simulink model "VbyFSpeedControl"  (R2017b)
settings: Solver=VariableStepAuto  StartTime=0.0  StopTime=10  MaxStep=1e-4  RelTol=1e-3
undefined symbols (not defined in the file): sigbuilder_block
libraries: powerlib x7, powerlib_meascontrol x1
settings Model: Creator=u4eee15106  LastModifiedBy=india
settings OptimizationCC: LifeSpan=inf
settings DebuggingCC: SFExecutionAtInitializationDiag=none
settings CodeAppCC: StateflowObjectComments=on

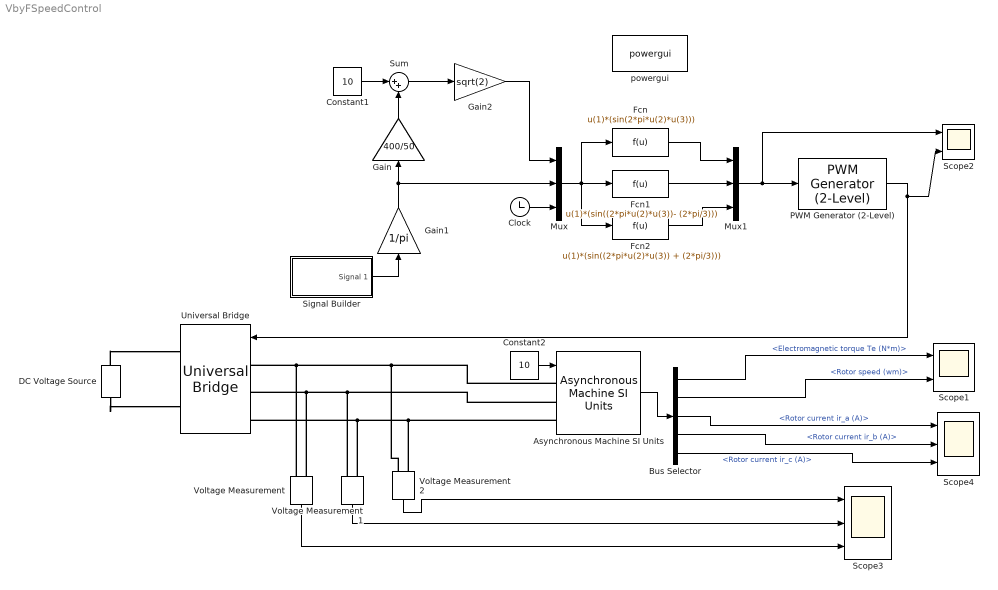
== system VbyFSpeedControl ==
  Asynchronous Machine SI Units : powerlib/Machines/Asynchronous Machine SI Units  RotorType=Squirrel-cage  PresetModel="15:  5.4 HP (4KW)   400 V  50Hz 1430 RPM"  MechanicalLoad=Torque Tm  ShowDetailedParameters=on  ReferenceFrame=Rotor  Units=SI  MeasurementBus=off  NominalParameters=[4000 400 50]  Stator=[1.405 0.005839]  Rotor=[1.395 0.005839]  Cage1=[0.4155 0.002066]  Cage2=[0.4168 0.0003495]  Lm=0.1722  Mechanical=[0.0131 0.002985 2]  PolePairs=2  InitialConditions=[0 0 0 0 0 0 0 0]  SimulateSaturation=off  Saturation=[14.03593122, 27.81365428, 53.79336849, 72.68890987, 97.98006896, 148.6815601, 215.7428561, 302.9841135, 428.7778367 ; 230, 322, 414, 460, 506, 552, 598, 644, 690]  LoadFlowParameters=1492000  TsPowergui=0  TsBlock=-1  IterativeModel=Trapezoidal non iterative  IterativeDiscreteModel=Trapezoidal non iterative  Pmec=1.492e+006
  Bus Selector : BusSelector  OutputSignals=Mechanical.Electromagnetic torque Te (N*m),Mechanical.Rotor speed (wm),Rotor measurements.Rotor current ir_a (A),Rotor measurements.Rotor current ir_b (A),Rotor measurements.Rotor current ir_c (A)
  Clock : Clock
  Constant1 : Constant  Value=10
  Constant2 : Constant  Value=10
  DC Voltage Source : powerlib/Electrical Sources/DC Voltage Source  Amplitude=415  Measurements=None
  Fcn : Fcn  Expr=u(1)*(sin(2*pi*u(2)*u(3)))
  Fcn1 : Fcn  Expr=u(1)*(sin((2*pi*u(2)*u(3))- (2*pi/3)))
  Fcn2 : Fcn  Expr=u(1)*(sin((2*pi*u(2)*u(3)) + (2*pi/3)))
  Gain : Gain  Gain=400/50
  Gain1 : Gain  Gain=1/pi
  Gain2 : Gain  Gain=sqrt(2)
  Mux : Mux  Inputs=3
  Mux1 : Mux  Inputs=3
  PWM Generator (2-Level) : powerlib_meascontrol/Pulse & Signal Generators/PWM Generator (2-Level)  ModulatorType=Three-phase bridge (6 pulses)  ModulatorMode=Unsynchronized  Fc=27*50  Pc=90  nF=27  MinMax="[ -1  1 ]"  SamplingTechnique=Natural  ModulatingSignals=off  m=0.8  Freq=60  Phase=0  Ts=0  ShowCarrierOutport=off
      settings: SourceProductName=Simscape Power Systems
  Scope1 : Scope  NumInputPorts=2
  Scope2 : Scope  NumInputPorts=2
  Scope3 : Scope  NumInputPorts=3
  Scope4 : Scope  NumInputPorts=3
  Signal Builder : Subsystem  Tag=STV Subsys  LoadFcn=sigbuilder_block('load');  StartFcn=sigbuilder_block('start');  StopFcn=sigbuilder_block('stop');  ClipboardFcn=sigbuilder_block('clipboard');  mask(Sigbuilder block){tuvar=[0:10]}
      mask help: Simulink:masks:SigbuilderBlock_MD
      mask init:
      | if ~strcmp(get_param(bdroot(gcbh),'SimulationStatus'),'stopped') tuvar = sigbuilder_block('maskInit'); end
      settings: CopyFcn=sigbuilder_block('copy');  DeleteFcn=sigbuilder_block('delete');  ModelCloseFcn=sigbuilder_block('modelClose');  PreSaveFcn=sigbuilder_block('preSave');  PauseFcn=sigbuilder_block('pause');  ContinueFcn=sigbuilder_block('continue');  NameChangeFcn=sigbuilder_block('namechange');  OpenFcn=sigbuilder_block('open',[5.4 5.4 1141.2 580.8 ]);  CloseFcn=sigbuilder_block('close');
      mask Display: plot(0, 0, 100, 100,[2, 2, 32, 32, 2], [68, 8, 8, 68, 68],[32, 2], [38, 38], [32, 19, 2],[53, 60, 44], [32, 17, 17, 2],[16, 16, 31, 31]);txt = getActiveGroup(gcbh);text(2, 100, txt,'verticalAlignment', 'top');
  Sum : Sum  Inputs=|++
  Universal Bridge : powerlib/Power Electronics/Universal Bridge  Arms=3  SnubberResistance=1e5  SnubberCapacitance=inf  Device=MOSFET / Diodes  Ron=1e-3  Lon=0  ForwardVoltages="[  0  0  ]"  ForwardVoltage=0  GTOparameters=[ 10e-6 , 20e-6 ]  IGBTparameters=[ 1e-6 , 2e-6 ]  Measurements=None  Measurements_2=None  converterType=Rectifier
  Voltage Measurement : powerlib/Measurements/Voltage Measurement  PhasorSimulation=off  OutputType=Complex  PSBequivalent=0
  Voltage Measurement1 : powerlib/Measurements/Voltage Measurement  PhasorSimulation=off  OutputType=Complex  PSBequivalent=0
  Voltage Measurement2 : powerlib/Measurements/Voltage Measurement  PhasorSimulation=off  OutputType=Complex  PSBequivalent=0
  powergui : powerlib/powergui  Priority=1  SimulationMode=Continuous  SampleTime=50e-6  frequency=60  Iterations=50  frequencyindice=50  Pbase=100e6  ErrMax=1e-4  UnitsV=kV  UnitsW=MW  buscounter=0  FunctionMessages=off  echomessages=off  EnableUseOfTLC=off  CurrentSourceSwitches=off  DisableSnubberDevices=off  DisableRonSwitches=off  DisableVfSwitches=off  DisplayEquations=off  SolverType=Tustin/Backward Euler (TBE)  Interpol=off  ExternalGateDelay=off  methode=off  Ts=100  x0status=blocks  SPID=on  SwTol=0  HookPort=off  RestoreLinks=warning  ResistiveCurrentMeasurement=off  Frange=[0:2:500]  Ylog=off  Xlog=on  ShowGrid=off  save=off  variable=ZData  structure=0  ZoomFFT=off  StartTime=0.0  cycles=1  DisplayStyle=1  fundamental=60  FreqAxis=off  MaxFrequency=1000  frequencyindicesteady=1  RmsSteady=1  display=off
  wires:
  Mux/1 -> Fcn2/1, Fcn1/1, Fcn/1
  Gain/1 -> Sum/2
  Gain1/1 -> Mux/2, Gain/1
  Clock/1 -> Mux/3
  Mux1/1 -> PWM Generator (2-Level)/1, Scope2/1
  PWM Generator (2-Level)/1 -> Scope2/2, Universal Bridge/1
  Constant1/1 -> Sum/1
  Asynchronous Machine SI Units/1 -> Bus Selector/1
  Bus Selector/2 -> Scope1/2  "<Rotor speed (wm)>"
  Bus Selector/1 -> Scope1/1  "<Electromagnetic torque Te (N*m)>"
  Sum/1 -> Gain2/1
  Gain2/1 -> Mux/1
  Fcn1/1 -> Mux1/2
  Fcn/1 -> Mux1/1
  Fcn2/1 -> Mux1/3
  Constant2/1 -> Asynchronous Machine SI Units/1
  Signal Builder/1(Signal 1) -> Gain1/1
  Voltage Measurement/1 -> Scope3/3
  Voltage Measurement1/1 -> Scope3/2
  Voltage Measurement2/1 -> Scope3/1
  Bus Selector/3 -> Scope4/1  "<Rotor current ir_a (A)>"
  Bus Selector/4 -> Scope4/2  "<Rotor current ir_b (A)>"
  Bus Selector/5 -> Scope4/3  "<Rotor current ir_c (A)>"
  connections:
  Asynchronous Machine SI Units/LConn3 -- Voltage Measurement2/LConn1 -- Voltage Measurement1/LConn2 -- Universal Bridge/LConn3
  Asynchronous Machine SI Units/LConn2 -- Voltage Measurement1/LConn1 -- Voltage Measurement/LConn2 -- Universal Bridge/LConn2
  Asynchronous Machine SI Units/LConn1 -- Voltage Measurement2/LConn2 -- Voltage Measurement/LConn1 -- Universal Bridge/LConn1
  DC Voltage Source/RConn1 -- Universal Bridge/RConn1
  DC Voltage Source/LConn1 -- Universal Bridge/RConn2

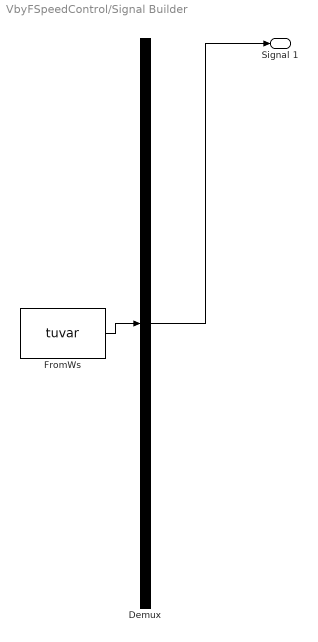
== system VbyFSpeedControl/Signal Builder ==
  Demux : Demux  Tag=STV Demux  Outputs=1
  FromWs : FromWorkspace  Tag=STV FromWs  VariableName=tuvar  SampleTime=0
      SigBuilderData=|
      | common.afterFinalStr = 'Extrapolate'
      | common.sampleTime = 0
      | dataSet.timeRange = [0 10]
      | dataSet.name = 'Group 1'
      | sbobj.Groups.Name = 'Group 1'
      | sbobj.Groups.Signals.Name = 'Signal 1'
      | sbobj.Groups.Signals.XData = [0 1 1 2 3 3 4 5 5 6 7 7 8.02 9 9 10]
      | sbobj.Groups.Signals.YData = [0 0 40 40 40 80 80 80 120 120 120 160 160 160 200 200]
  Signal 1 : Outport  Tag=STV Outport
  wires:
  Demux/1 -> Signal 1/1
  FromWs/1 -> Demux/1
